simulink model "RflysimIndoorController_r2018b_N12_V9"  (R2018b)
settings: Solver=ode4  StartTime=0.0  StopTime=inf  FixedStep=ts  MaxStep=0.6  RelTol=1e-3
values from neighbouring files (symbols this model uses):
  l_v = 5    [RflyMain.m]    (also in RflyMain_N12_V6.m; RflyMain_N6_V3.m; RflyMain_N6_V4.m; RflyMain_V2.m)
  p_target = [200,10]    [RflyMain.m]    (also in RflyMain_N12_V6.m; RflyMain_N6_V3.m; RflyMain_N6_V4.m; RflyMain_V2.m)
  ra = 0.6    [RflyMain.m]    (also in RflyMain_N12_V6.m; RflyMain_N6_V3.m; RflyMain_N6_V4.m; RflyMain_V2.m)
  rs = 0.25    [RflyMain.m]    (also in RflyMain_N12_V6.m; RflyMain_N6_V3.m; RflyMain_N6_V4.m; RflyMain_V2.m)
  rt_a = 1.5    [RflyMain_N12_V6.m]
  rt_s = 0.25    [RflyMain_N12_V6.m]
  ts = [0 0]    [QuadModel2D.m]    (also in RflyMain.m = 0.01; RflyMain_N12_V6.m = 0.05; RflyMain_N6_V3.m = 0.05; RflyMain_N6_V4.m = 0.05)
  v_max = 2    [RflyMain.m]    (also in RflyMain_N12_V6.m = 3; RflyMain_N6_V3.m = 3; RflyMain_N6_V4.m = 3; RflyMain_V2.m = 3)
undefined symbols (not defined in the file or in its folder): Twist
libraries: robotlib x96, aerolibanimutils x1
(part 2 of 2)

== matlab function RflysimIndoorController_r2018b_N12_V9/MATLAB Function2 ==
  data: states input; tunnel_msg1 input; tunnel_msg2 input; tunnel_msg3 input; tunnel_msg4 input; tunnel_msg5 input; tunnel_msg6 input; tunnel_msg7 input; tunnel_msg8 input; tunnel_msg9 input; tunnel_msg10 input; tunnel_msg11 input; tunnel_msg12 input; ux output; uy output; uz output; p_target input; Pcur input; Vcur input; Zcur input; Yawcur input; gain input; vmax input; uyaw output; rs input; ra input; states_new output; p_radius output; p_left_encircle output; p_right_encircle output; rt1 input; rt2 input
function [ux,uy,uz,uyaw,states_new,p_radius,p_left_encircle,p_right_encircle]  = mytunnel(states,tunnel_msg1,tunnel_msg2,tunnel_msg3,tunnel_msg4,tunnel_msg5,tunnel_msg6,tunnel_msg7,tunnel_msg8,tunnel_msg9,tunnel_msg10,tunnel_msg11,tunnel_msg12,p_target,Pcur,Vcur,Zcur,Yawcur,gain,vmax,rs,ra,rt1,rt2)
p_target=p_target';

N=12;
ux=zeros(N,1);
uy=zeros(N,1);
uz=zeros(N,1);
uyaw=zeros(N,1);
states_new=zeros(N,1);
tunnel_msg=tunnel_msg1;
height_desire=4;

for j=1:N
    uz(j)=mysatNum((height_desire-Zcur(j))*0.8,-2,2);
    
    left_x=zeros(10,1);
    left_y=zeros(10,1);
    right_x=zeros(10,1);
    right_y=zeros(10,1);
    middle_x=zeros(10,1);
    middle_y=zeros(10,1);
    if j==1
        tunnel_msg=tunnel_msg1;
    elseif j==2
        tunnel_msg=tunnel_msg2;
    elseif j==3
        tunnel_msg=tunnel_msg3;
    elseif j==4
        tunnel_msg=tunnel_msg4;
    elseif j==5
        tunnel_msg=tunnel_msg5;
    elseif j==6
        tunnel_msg=tunnel_msg6;
    elseif j==7
        tunnel_msg=tunnel_msg7;
    elseif j==8
        tunnel_msg=tunnel_msg8;
    elseif j==9
        tunnel_msg=tunnel_msg9;
    elseif j==10
        tunnel_msg=tunnel_msg10;
    elseif j==11
        tunnel_msg=tunnel_msg11;
    elseif j==12
        tunnel_msg=tunnel_msg12;
    end
    tunnel_type = tunnel_msg.Pipetype.Data;
    point_num=tunnel_msg.Units_SL_Info.CurrentLength;
    
    for k=1:point_num
        left_x(k,1) = tunnel_msg.Units(k).Left.X;
        left_y(k,1) = tunnel_msg.Units(k).Left.Y;
        
        right_x(k,1) = tunnel_msg.Units(k).Right.X;
        right_y(k,1) = tunnel_msg.Units(k).Right.Y;
        
        middle_x(k,1) = tunnel_msg.Units(k).Middle.X;
        middle_y(k,1) = tunnel_msg.Units(k).Middle.Y;
    end
    
    left_x=left_x(1:point_num,1);
    left_y=left_y(1:point_num,1);
    right_x=right_x(1:point_num,1);
    right_y=right_y(1:point_num,1);
    middle_x=middle_x(1:point_num,1);
    middle_y=middle_y(1:point_num,1);
    
    inter_num = 500;
    p_radius=zeros(inter_num,2);
    p_left_encircle=zeros(inter_num,2);
    p_right_encircle=zeros(inter_num,2);
    
    if tunnel_type==10
        k=1:length(middle_x);
        ki=linspace(1,length(middle_x),inter_num); %%%%% 插值的点越多，控制更精确，曲线更光滑，计算更耗时
        p_radius_x=(interp1(k,middle_x,ki,'linear'))';
        p_radius_y=(interp1(k,middle_y,ki,'linear'))';
        p_radius(:,1)=p_radius_x;
        p_radius(:,2)=p_radius_y;
        
        k=1:length(left_x);
        ki=linspace(1,length(left_x),inter_num); %%%%% 插值的点越多，控制更精确，曲线更光滑，计算更耗时
        p_left_encircle_x=(interp1(k,left_x,ki,'linear'))';
        p_left_encircle_y=(interp1(k,left_y,ki,'linear'))';

        p_left_encircle(:,1)=p_left_encircle_x;
        p_left_encircle(:,2)=p_left_encircle_y;
        
        k=1:length(right_x);
        ki=linspace(1,length(right_x),inter_num); %%%%% 插值的点越多，控制更精确，曲线更光滑，计算更耗时
        p_right_encircle_x=(interp1(k,right_x,ki,'linear'))';
        p_right_encircle_y=(interp1(k,right_y,ki,'linear'))';
        p_right_encircle(:,1)=p_right_encircle_x;
        p_right_encircle(:,2)=p_right_encircle_y;
    end
    
    
    
    [u_encircle,ux_encircle,uy_encircle,uyaw_encircle,leader_locate,dist_encircle]  = Encirclement4(p_radius,p_left_encircle,p_right_encircle,p_target,Pcur,Vcur,Yawcur,gain,vmax,rs,ra,rt1,rt2,j);
    
    if states(j)==30
        states_new(j)=30;
        if tunnel_type==10
            ux(j)=ux_encircle;
            uy(j)=uy_encircle;
            uyaw(j)=uyaw_encircle;
            if abs(leader_locate-inter_num)<5
                states_new(j)=20;
            end
        end
    end
end

== matlab function RflysimIndoorController_r2018b_N12_V9/Position, Yaw and Velocity/MATLAB Function ==
  data: u input; yaw output
function yaw = fcn(u)
q0=u.W;
q1=u.X;
q2=u.Y;
q3=u.Z;
yaw = atan2(2*(q0*q3+q1*q2), 1-2*(q2*q2+q3*q3));

== matlab function RflysimIndoorController_r2018b_N12_V9/MATLAB Function3 ==
  data: state input; tri1 output; tri2 output; tri3 output; tri4 output; tri5 output; tri6 output; tri7 output; tri8 output; tri9 output; tri10 output; tri11 output; tri12 output
function [tri1,tri2,tri3,tri4,tri5,tri6,tri7,tri8,tri9,tri10,tri11,tri12] = fcn(state)
tri1=0;
tri2=0;
tri3=0;
tri4=0;
tri5=0;
tri6=0;
tri7=0;
tri8=0;
tri9=0;
tri10=0;
tri11=0;
tri12=0;
if state(1)==30
    tri1=1;
end
if state(2)==30
    tri2=1;
end
if state(3)==30
    tri3=1;
end
if state(4)==30
    tri4=1;
end
if state(5)==30
    tri5=1;
end
if state(6)==30
    tri6=1;
end
if state(7)==30
    tri7=1;
end
if state(8)==30
    tri8=1;
end
if state(9)==30
    tri9=1;
end
if state(10)==30
    tri10=1;
end
if state(11)==30
    tri11=1;
end
if state(12)==30
    tri12=1;
end

== matlab function RflysimIndoorController_r2018b_N12_V9/MATLAB Function4 ==
  data: msg input; msg_new output Bus_type; msg_last input
function msg_new = fcn(msg,msg_last)
if msg.Units_SL_Info.CurrentLength==0
    msg_new=msg_last;
else
    msg_new=msg;
end

== matlab function RflysimIndoorController_r2018b_N12_V9/MATLAB Function5 ==
  data: msg input; msg_new output Bus_type; msg_last input
function msg_new = fcn(msg,msg_last)
if msg.Units_SL_Info.CurrentLength==0
    msg_new=msg_last;
else
    msg_new=msg;
end

== matlab function RflysimIndoorController_r2018b_N12_V9/MATLAB Function6 ==
  data: msg input; msg_new output Bus_type; msg_last input
function msg_new = fcn(msg,msg_last)
if msg.Units_SL_Info.CurrentLength==0
    msg_new=msg_last;
else
    msg_new=msg;
end

== matlab function RflysimIndoorController_r2018b_N12_V9/Position, Yaw and Velocity/MATLAB Function7 ==
  data: u input; yaw output
function yaw = fcn(u)
q0=u.W;
q1=u.X;
q2=u.Y;
q3=u.Z;
yaw = atan2(2*(q0*q3+q1*q2), 1-2*(q2*q2+q3*q3));

== matlab function RflysimIndoorController_r2018b_N12_V9/MATLAB Function8 ==
  data: msg input; msg_new output Bus_type; msg_last input
function msg_new = fcn(msg,msg_last)
if msg.Units_SL_Info.CurrentLength==0
    msg_new=msg_last;
else
    msg_new=msg;
end

== matlab function RflysimIndoorController_r2018b_N12_V9/MATLAB Function10 ==
  data: msg input; msg_new output Bus_type; msg_last input
function msg_new = fcn(msg,msg_last)
if msg.Units_SL_Info.CurrentLength==0
    msg_new=msg_last;
else
    msg_new=msg;
end

== matlab function RflysimIndoorController_r2018b_N12_V9/Position, Yaw and Velocity/MATLAB Function9 ==
  data: u input; yaw output
function yaw = fcn(u)
q0=u.W;
q1=u.X;
q2=u.Y;
q3=u.Z;
yaw = atan2(2*(q0*q3+q1*q2), 1-2*(q2*q2+q3*q3));

== matlab function RflysimIndoorController_r2018b_N12_V9/Position, Yaw and Velocity/MATLAB Function11 ==
  data: x1 input; Pcur output; y1 input; x2 input; y2 input; x3 input; y3 input; x4 input; y4 input; x5 input; y5 input; x6 input; y6 input; x7 input; y7 input; x8 input; y8 input; x9 input; y9 input; x10 input; y10 input; x11 input; y11 input; x12 input; y12 input
function Pcur = fcn(x1,y1,x2,y2,x3,y3,x4,y4,x5,y5,x6,y6,x7,y7,x8,y8,x9,y9,x10,y10,x11,y11,x12,y12)
Pcur=[x1,y1;x2,y2;x3,y3;x4,y4;x5,y5;x6,y6;x7,y7;x8,y8;x9,y9;x10,y10;x11,y11;x12,y12];

== matlab function RflysimIndoorController_r2018b_N12_V9/Position, Yaw and Velocity/MATLAB Function12 ==
  data: x1 input; Vcur output; y1 input; x2 input; y2 input; x3 input; y3 input; x4 input; y4 input; x5 input; y5 input; x6 input; y6 input; x7 input; y7 input; x8 input; y8 input; x9 input; y9 input; x10 input; y10 input; x11 input; y11 input; x12 input; y12 input
function Vcur = fcn(x1,y1,x2,y2,x3,y3,x4,y4,x5,y5,x6,y6,x7,y7,x8,y8,x9,y9,x10,y10,x11,y11,x12,y12)
Vcur=[x1,y1;x2,y2;x3,y3;x4,y4;x5,y5;x6,y6;x7,y7;x8,y8;x9,y9;x10,y10;x11,y11;x12,y12];

== matlab function RflysimIndoorController_r2018b_N12_V9/MATLAB Function7 ==
  data: msg input; msg_new output Bus_type; msg_last input
function msg_new = fcn(msg,msg_last)
if msg.Units_SL_Info.CurrentLength==0
    msg_new=msg_last;
else
    msg_new=msg;
end

== matlab function RflysimIndoorController_r2018b_N12_V9/Position, Yaw and Velocity/MATLAB Function1 ==
  data: u input; yaw output
function yaw = fcn(u)
q0=u.W;
q1=u.X;
q2=u.Y;
q3=u.Z;
yaw = atan2(2*(q0*q3+q1*q2), 1-2*(q2*q2+q3*q3));

== matlab function RflysimIndoorController_r2018b_N12_V9/Position, Yaw and Velocity/MATLAB Function2 ==
  data: u input; yaw output
function yaw = fcn(u)
q0=u.W;
q1=u.X;
q2=u.Y;
q3=u.Z;
yaw = atan2(2*(q0*q3+q1*q2), 1-2*(q2*q2+q3*q3));

== matlab function RflysimIndoorController_r2018b_N12_V9/Position, Yaw and Velocity/MATLAB Function3 ==
  data: u input; yaw output
function yaw = fcn(u)
q0=u.W;
q1=u.X;
q2=u.Y;
q3=u.Z;
yaw = atan2(2*(q0*q3+q1*q2), 1-2*(q2*q2+q3*q3));

== matlab function RflysimIndoorController_r2018b_N12_V9/MATLAB Function11 ==
  data: msg input; msg_new output Bus_type; msg_last input
function msg_new = fcn(msg,msg_last)
if msg.Units_SL_Info.CurrentLength==0
    msg_new=msg_last;
else
    msg_new=msg;
end

== matlab function RflysimIndoorController_r2018b_N12_V9/MATLAB Function12 ==
  data: msg input; msg_new output Bus_type; msg_last input
function msg_new = fcn(msg,msg_last)
if msg.Units_SL_Info.CurrentLength==0
    msg_new=msg_last;
else
    msg_new=msg;
end

== matlab function RflysimIndoorController_r2018b_N12_V9/MATLAB Function13 ==
  data: msg input; msg_new output Bus_type; msg_last input
function msg_new = fcn(msg,msg_last)
if msg.Units_SL_Info.CurrentLength==0
    msg_new=msg_last;
else
    msg_new=msg;
end

== matlab function RflysimIndoorController_r2018b_N12_V9/MATLAB Function14 ==
  data: msg input; msg_new output Bus_type; msg_last input
function msg_new = fcn(msg,msg_last)
if msg.Units_SL_Info.CurrentLength==0
    msg_new=msg_last;
else
    msg_new=msg;
end

== matlab function RflysimIndoorController_r2018b_N12_V9/MATLAB Function15 ==
  data: msg input; msg_new output Bus_type; msg_last input
function msg_new = fcn(msg,msg_last)
if msg.Units_SL_Info.CurrentLength==0
    msg_new=msg_last;
else
    msg_new=msg;
end

== matlab function RflysimIndoorController_r2018b_N12_V9/MATLAB Function9 ==
  data: msg input; msg_new output Bus_type; msg_last input
function msg_new = fcn(msg,msg_last)
if msg.Units_SL_Info.CurrentLength==0
    msg_new=msg_last;
else
    msg_new=msg;
end

== matlab function RflysimIndoorController_r2018b_N12_V9/Position, Yaw and Velocity/MATLAB Function10 ==
  data: u input; yaw output
function yaw = fcn(u)
q0=u.W;
q1=u.X;
q2=u.Y;
q3=u.Z;
yaw = atan2(2*(q0*q3+q1*q2), 1-2*(q2*q2+q3*q3));

== matlab function RflysimIndoorController_r2018b_N12_V9/Position, Yaw and Velocity/MATLAB Function13 ==
  data: u input; yaw output
function yaw = fcn(u)
q0=u.W;
q1=u.X;
q2=u.Y;
q3=u.Z;
yaw = atan2(2*(q0*q3+q1*q2), 1-2*(q2*q2+q3*q3));

== matlab function RflysimIndoorController_r2018b_N12_V9/Position, Yaw and Velocity/MATLAB Function4 ==
  data: u input; yaw output
function yaw = fcn(u)
q0=u.W;
q1=u.X;
q2=u.Y;
q3=u.Z;
yaw = atan2(2*(q0*q3+q1*q2), 1-2*(q2*q2+q3*q3));

== matlab function RflysimIndoorController_r2018b_N12_V9/Position, Yaw and Velocity/MATLAB Function5 ==
  data: u input; yaw output
function yaw = fcn(u)
q0=u.W;
q1=u.X;
q2=u.Y;
q3=u.Z;
yaw = atan2(2*(q0*q3+q1*q2), 1-2*(q2*q2+q3*q3));

== matlab function RflysimIndoorController_r2018b_N12_V9/Position, Yaw and Velocity/MATLAB Function6 ==
  data: u input; yaw output
function yaw = fcn(u)
q0=u.W;
q1=u.X;
q2=u.Y;
q3=u.Z;
yaw = atan2(2*(q0*q3+q1*q2), 1-2*(q2*q2+q3*q3));

== matlab function RflysimIndoorController_r2018b_N12_V9/Position, Yaw and Velocity/MATLAB Function8 ==
  data: u input; yaw output
function yaw = fcn(u)
q0=u.W;
q1=u.X;
q2=u.Y;
q3=u.Z;
yaw = atan2(2*(q0*q3+q1*q2), 1-2*(q2*q2+q3*q3));
